simulink model "Copy_of_MRStandardSimulation"  (R2021a)
settings: Solver=VariableStepAuto  StartTime=0.0  StopTime=t(end)  RelTol=1e-3
values from neighbouring files (symbols this model uses):
  F = 10    [MRStandardPlantLPMExample.m]
  J = [   0  0 0 1 ... (first row only)    [MRStandardPlantLPMExample.m]
  Kd = c2d(K,TsL)    [MRStandardPlantLPMExample.m]    (also in SIMOLPMTest.m = c2d(ss(K),Ts))
  L = Dscale\L    [MRLPMClosedLoopFastBLA2.m]    (also in MRLPMClosedLoopFastBLAWeighted.m; MRLPMOpenLoopFastBLA.m; MRLPMOpenLoopFastBLA2.m)
  Pd = c2d(P,TsH)    [MRStandardPlantLPMExample.m]    (also in SIMOLPMTest.m = c2d(P,Ts,'zoh'))
  rH = repmat(rH,per,1)    [MRStandardPlantLPMExample.m]    (also in MultiRateLPM.m = repmat(rp,Per,1))
  TsH = 1/fs    (= 0.004)    [MRStandardPlantLPMExample.m]    (also in MultiRateLPM.m = 0.005; MultiratePFG.m = 0.005; unliftfrd.m = TsL/F; unliftfrdWithoutRep.m = GliftSIMO.Ts)
  TsL = 1/fsL    (= 0.04)    [MRStandardPlantLPMExample.m]    (also in MultiRateLPM.m = 0.01; MultiratePFG.m = 0.01; unliftfrd.m = GliftSIMO.Ts)
libraries: simulink x1, dspsrcs4 x1
settings Model: Creator=s152009  LastModifiedBy=s152009
settings DebuggingCC: AlgebraicLoopMsg=none

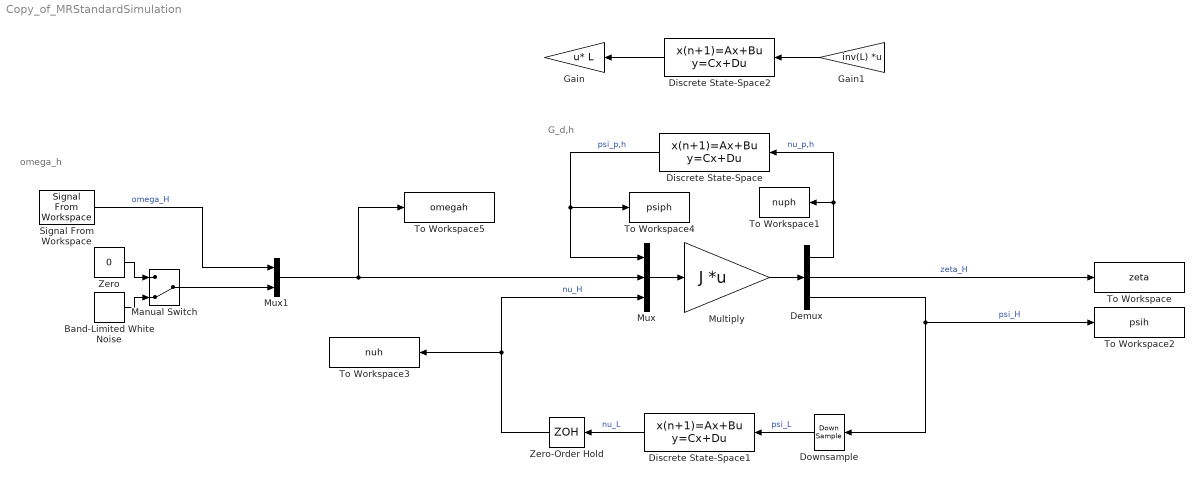
== system Copy_of_MRStandardSimulation ==
  note: omega_h
  note: G_d,h
  Band-Limited White Noise : simulink/Sources/Band-Limited White Noise  Cov=0.000005  Ts=TsH  seed=[23341]
  Demux : Demux  Outputs=3
  Discrete State-Space : DiscreteStateSpace  A=ss(Pd).A  B=ss(Pd).B  C=ss(Pd).C  D=ss(Pd).D  SampleTime=TsH
  Discrete State-Space1 : DiscreteStateSpace  A=ss(Kd).A  B=ss(Kd).B  C=ss(Kd).C  D=ss(Kd).D  SampleTime=TsL
  Discrete State-Space2 : DiscreteStateSpace  A=ss(Pd).A  B=ss(Pd).B  C=ss(Pd).C  D=ss(Pd).D  SampleTime=TsH
  Downsample : DownSample  N=F  RateOptions=Allow multirate processing
  Gain : Gain  Gain=L  Multiplication=Matrix(u*K)
  Gain1 : Gain  Gain=inv(L)  Multiplication=Matrix(K*u)
  Manual Switch : ManualSwitch  CurrentSetting=0
  Multiply : Gain  Gain=J  Multiplication=Matrix(K*u) (u vector)
  Mux : Mux  Inputs=3
  Mux1 : Mux  Inputs=2
  Signal From Workspace : dspsrcs4/Signal From Workspace  X=real(rH)  Ts=TsH  nsamps=1  OutputAfterFinalValue=Setting to zero  ignoreOrWarnInputAndFrameLengths=off  OutputFrames=off
  To Workspace : ToWorkspace  VariableName=zeta  SampleTime=TsH
      settings: Save2DSignal=2-D array (concatenate along first dimension)
  To Workspace1 : ToWorkspace  VariableName=nuph  SampleTime=TsH
      settings: Save2DSignal=2-D array (concatenate along first dimension)
  To Workspace2 : ToWorkspace  VariableName=psih  SampleTime=TsH
      settings: Save2DSignal=2-D array (concatenate along first dimension)
  To Workspace3 : ToWorkspace  VariableName=nuh  SampleTime=TsH
      settings: Save2DSignal=2-D array (concatenate along first dimension)
  To Workspace4 : ToWorkspace  VariableName=psiph  SampleTime=TsH
      settings: Save2DSignal=2-D array (concatenate along first dimension)
  To Workspace5 : ToWorkspace  VariableName=omegah  SampleTime=TsH
      settings: Save2DSignal=2-D array (concatenate along first dimension)
  Zero : Constant  Value=0  OutDataTypeStr=Inherit: Inherit via back propagation
  Zero-Order Hold : ZeroOrderHold  SampleTime=TsH
  wires:
  Mux/1 -> Multiply/1
  Multiply/1 -> Demux/1
  Demux/1 -> Discrete State-Space/1, To Workspace1/1  "nu_p,h"
  Zero-Order Hold/1 -> Mux/3, To Workspace3/1  "nu_H"
  Demux/3 -> To Workspace2/1, Downsample/1  "psi_H"
  Downsample/1 -> Discrete State-Space1/1  "psi_L"
  Discrete State-Space1/1 -> Zero-Order Hold/1  "nu_L"
  Demux/2 -> To Workspace/1  "zeta_H"
  Discrete State-Space/1 -> To Workspace4/1, Mux/1  "psi_p,h"
  Signal From Workspace/1 -> Mux1/1  "omega_H"
  Manual Switch/1 -> Mux1/2
  Band-Limited White Noise/1 -> Manual Switch/2
  Zero/1 -> Manual Switch/1
  Mux1/1 -> To Workspace5/1, Mux/2
  Discrete State-Space2/1 -> Gain/1
  Gain1/1 -> Discrete State-Space2/1
